simulink model "Controller_HIL"  (R2023b)
settings: Solver=FixedStepDiscrete  StartTime=0.0  StopTime=inf  FixedStep=ts_controller  RelTol=1e-3
InitFcn:
  | mbd_s32k_consistency_checks(bdroot(gcs));
undefined symbols (not defined in the file): Battery, BMS_Controller_State, Charging_State, currentFactor, CV_Gain, DiscIntNeverNeededParam, I_cc, LQFP, MaxCellVoltThrsld, noCurrent, Ns_Module, NumModules, OverCellVoltageLimit, SOCInit, SRE, ts_controller, ts_system, UnderCellVoltageLimit, voltThreshold
libraries: mbd_s32k1xx_ec_toolbox x20, mbd_bcc_ec_toolbox x16, etargetslib x11, simulink x5, sharedTrackingLibrary x2, hdlsllib x1
(part 2 of 2)

== system Controller_HIL/Controller/Controller/SOC Calculation/Measurement Function ==
  Current : Inport
  Temperature (K) : Inport  Port=2
  batteryMeasurementFcn : TriggerPort  TriggerType=function-call  IsSimulinkFunction=on  FunctionName=batteryMeasurementFcn  VariantControl=Variant
  Add1 : Sum  Inputs=+--
  Em Table : Lookup_n-D  BreakpointsForDimension1=Battery.SOC_LUT  BreakpointsForDimension2=Battery.Temperature_LUT  BeginIndexSearchUsingPreviousIndexResult=on  Table=Battery.Em_LUT  ExtrapMethod=Clip  InternalRulePriority=Speed  RndMeth=Simplest
      settings: InputPortMap=u0,u1
  Get SOC : Selector  InputPortWidth=2  IndexOptions=Index vector (dialog)  Indices=[1]  OutputSizes=1
  Get U1 : Selector  InputPortWidth=2  IndexOptions=Index vector (dialog)  Indices=2  OutputSizes=1
  Product : Product
  R0 Table : Lookup_n-D  BreakpointsForDimension1=Battery.SOC_LUT  BreakpointsForDimension2=Battery.Temperature_LUT  BeginIndexSearchUsingPreviousIndexResult=on  Table=Battery.R0_LUT  ExtrapMethod=Clip  InternalRulePriority=Speed  RndMeth=Simplest
      settings: InputPortMap=u0,u1
  x : ArgIn  DisableCoverage=on  OutDataTypeStr=single  PortDimensions=2  ArgumentName=x
  y : ArgOut  DisableCoverage=on  OutDataTypeStr=single  ArgumentName=y
  wires:
  Get U1/1 -> Add1/3  "U1"
  Product/1 -> Add1/2
  Current/1 -> Product/2
  R0 Table/1 -> Product/1
  Temperature (K)/1 -> Em Table/2, R0 Table/2
  Add1/1 -> y/1
  Em Table/1 -> Add1/1
  Get SOC/1 -> Em Table/1, R0 Table/1  "SOC"
  x/1 -> Get SOC/1, Get U1/1

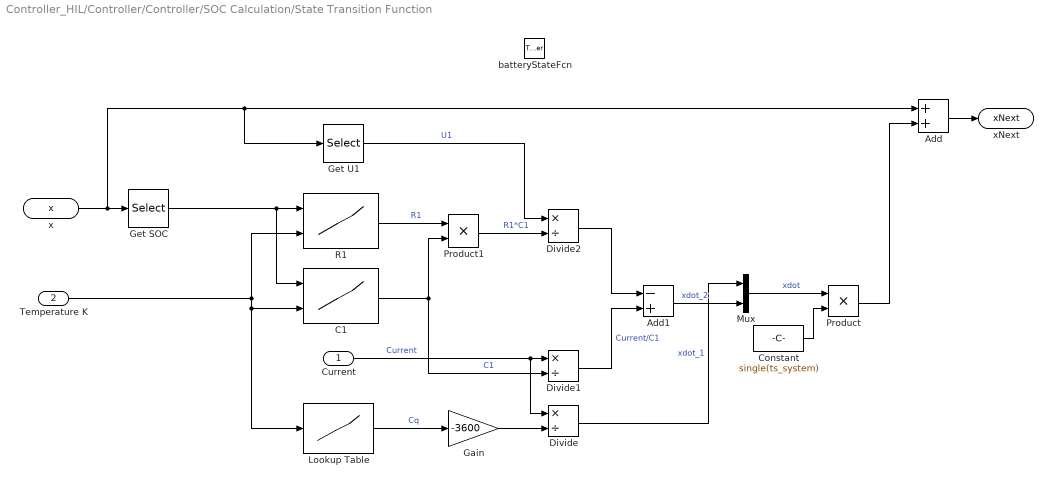
== system Controller_HIL/Controller/Controller/SOC Calculation/State Transition Function ==
  Current : Inport
  Temperature K : Inport  Port=2
  batteryStateFcn : TriggerPort  TriggerType=function-call  IsSimulinkFunction=on  FunctionName=batteryStateFcn  VariantControl=Variant
  Add : Sum
  Add1 : Sum  Inputs=-+
  C1 : Lookup_n-D  BreakpointsForDimension1=Battery.SOC_LUT  BreakpointsForDimension2=Battery.Temperature_LUT  BeginIndexSearchUsingPreviousIndexResult=on  Table=Battery.C1_LUT  ExtrapMethod=Clip  InternalRulePriority=Speed  RndMeth=Simplest
      settings: InputPortMap=u0,u1
  Constant : Constant  Value=single(ts_system)  OutDataTypeStr=single
  Divide : Product  Inputs=*/
  Divide1 : Product  Inputs=*/
  Divide2 : Product  Inputs=*/
  Gain : Gain  Gain=-3600
  Get SOC : Selector  InputPortWidth=2  IndexOptions=Index vector (dialog)  Indices=1  OutputSizes=1
  Get U1 : Selector  InputPortWidth=2  IndexOptions=Index vector (dialog)  Indices=2  OutputSizes=1
  Lookup Table : Lookup_n-D  NumberOfTableDimensions=1  BreakpointsForDimension1=Battery.Temperature_LUT  BeginIndexSearchUsingPreviousIndexResult=on  Table=Battery.Capacity_LUT  InternalRulePriority=Speed  RndMeth=Simplest
  Mux : Mux  Inputs=2
  Product : Product  OutDataTypeStr=single
  Product1 : Product
  R1 : Lookup_n-D  BreakpointsForDimension1=Battery.SOC_LUT  BreakpointsForDimension2=Battery.Temperature_LUT  BeginIndexSearchUsingPreviousIndexResult=on  Table=Battery.R1_LUT  ExtrapMethod=Clip  InternalRulePriority=Speed  RndMeth=Simplest
      settings: InputPortMap=u0,u1
  x : ArgIn  DisableCoverage=on  OutDataTypeStr=single  PortDimensions=2  ArgumentName=x
  xNext : ArgOut  DisableCoverage=on  OutDataTypeStr=single  PortDimensions=2  ArgumentName=xNext
  wires:
  Lookup Table/1 -> Gain/1  "Cq"
  Product/1 -> Add/2
  Constant/1 -> Product/2
  Current/1 -> Divide1/1, Divide/1  "Current"
  Get SOC/1 -> C1/1, R1/1
  Temperature K/1 -> Lookup Table/1, C1/2, R1/2
  Add/1 -> xNext/1
  x/1 -> Add/1, Get U1/1, Get SOC/1
  Gain/1 -> Divide/2
  Divide/1 -> Mux/1  "xdot_1"
  Get U1/1 -> Divide2/1  "U1"
  Product1/1 -> Divide2/2  "R1*C1"
  R1/1 -> Product1/1  "R1"
  C1/1 -> Product1/2, Divide1/2  "C1"
  Divide1/1 -> Add1/2  "Current/C1"
  Divide2/1 -> Add1/1
  Add1/1 -> Mux/2  "xdot_2"
  Mux/1 -> Product/1  "xdot"

== system Controller_HIL/Controller/Controller/SOC Calculation/UKF_EKF_1TC ==
  Cell_Voltage : Inport
  Enable : EnablePort
  EKF : sharedTrackingLibrary/Extended Kalman Filter  StateTransitionFcn=batteryStateFcn  HasStateTransitionJacobianFcn=off  HasAdditiveProcessNoise=Additive  ProcessNoise=1e-10*eye(2)  HasTimeVaryingProcessNoise=off  HasStateTransitionFcnExtraArgument=0  InitialState=[single(SOCInit+0.05); 0;]  InitialStateCovariance=[1e-5 1]  MeasurementFcn1=batteryMeasurementFcn  HasMeasurementJacobianFcn1=off  HasMeasurementEnablePort1=off  HasAdditiveMeasurementNoise1=Additive  MeasurementNoise1=1e-1  HasTimeVaryingMeasurementNoise1=off  HasMeasurementFcnExtraArgument1=0  HasMeasurementWrapping1=off  MeasurementFcn2=myMeasurementFcn  HasMeasurementJacobianFcn2=off  HasMeasurementEnablePort2=off  HasAdditiveMeasurementNoise2=Additive  MeasurementNoise2=1  HasTimeVaryingMeasurementNoise2=off  HasMeasurementFcnExtraArgument2=0  HasMeasurementWrapping2=off  MeasurementFcn3=myMeasurementFcn  HasMeasurementJacobianFcn3=off  HasMeasurementEnablePort3=off  HasAdditiveMeasurementNoise3=Additive  MeasurementNoise3=1  HasTimeVaryingMeasurementNoise3=off  HasMeasurementFcnExtraArgument3=0  HasMeasurementWrapping3=off  MeasurementFcn4=myMeasurementFcn  HasMeasurementJacobianFcn4=off  HasMeasurementEnablePort4=off  HasAdditiveMeasurementNoise4=Additive  MeasurementNoise4=1  HasTimeVaryingMeasurementNoise4=off  HasMeasurementFcnExtraArgument4=0  HasMeasurementWrapping4=off  MeasurementFcn5=myMeasurementFcn  HasMeasurementJacobianFcn5=off  HasMeasurementEnablePort5=off  HasAdditiveMeasurementNoise5=Additive  MeasurementNoise5=1  HasTimeVaryingMeasurementNoise5=off  HasMeasurementFcnExtraArgument5=0  HasMeasurementWrapping5=off  EnableMultirate=off  StateTransitionFcnSampleTime=1  MeasurementFcn1SampleTime=1  MeasurementFcn2SampleTime=1  MeasurementFcn3SampleTime=1  MeasurementFcn4SampleTime=1  MeasurementFcn5SampleTime=1  UseCurrentEstimator=on  OutputStateCovariance=off  DataType=single  SampleTime=ts_controller  NumberOfMeasurements=1
  SOC : Selector  InputPortWidth=2  IndexOptions=Index vector (dialog)  Indices=1  OutputSizes=1
  SOC1 : Selector  InputPortWidth=2  IndexOptions=Index vector (dialog)  Indices=1  OutputSizes=1
  UKF : sharedTrackingLibrary/Unscented Kalman Filter  StateTransitionFcn=batteryStateFcn  HasAdditiveProcessNoise=Additive  ProcessNoise=1e-10*eye(2)  HasTimeVaryingProcessNoise=off  HasStateTransitionFcnExtraArgument=0  InitialState=[single(SOCInit+0.05); 0;]  InitialStateCovariance=[1e-5 1]  Alpha=1  Beta=2  Kappa=1  MeasurementFcn1=batteryMeasurementFcn  HasMeasurementEnablePort1=off  HasAdditiveMeasurementNoise1=Additive  MeasurementNoise1=0.1  HasTimeVaryingMeasurementNoise1=off  HasMeasurementFcnExtraArgument1=0  HasMeasurementWrapping1=off  MeasurementFcn2=myMeasurementFcn  HasMeasurementEnablePort2=off  HasAdditiveMeasurementNoise2=Additive  MeasurementNoise2=1  HasTimeVaryingMeasurementNoise2=off  HasMeasurementFcnExtraArgument2=0  HasMeasurementWrapping2=off  MeasurementFcn3=myMeasurementFcn  HasMeasurementEnablePort3=off  HasAdditiveMeasurementNoise3=Additive  MeasurementNoise3=1  HasTimeVaryingMeasurementNoise3=off  HasMeasurementFcnExtraArgument3=0  HasMeasurementWrapping3=off  MeasurementFcn4=myMeasurementFcn  HasMeasurementEnablePort4=off  HasAdditiveMeasurementNoise4=Additive  MeasurementNoise4=1  HasTimeVaryingMeasurementNoise4=off  HasMeasurementFcnExtraArgument4=0  HasMeasurementWrapping4=off  MeasurementFcn5=myMeasurementFcn  HasMeasurementEnablePort5=off  HasAdditiveMeasurementNoise5=Additive  MeasurementNoise5=1  HasTimeVaryingMeasurementNoise5=off  HasMeasurementFcnExtraArgument5=0  HasMeasurementWrapping5=off  EnableMultirate=off  StateTransitionFcnSampleTime=-1  MeasurementFcn1SampleTime=-1  MeasurementFcn2SampleTime=-1  MeasurementFcn3SampleTime=-1  MeasurementFcn4SampleTime=-1  MeasurementFcn5SampleTime=-1  UseCurrentEstimator=on  OutputStateCovariance=off  DataType=single  SampleTime=ts_controller  NumberOfMeasurements=1
  SOC_UKF : Outport  VectorParamsAs1DForOutWhenUnconnected=off
  SOC_EKF : Outport  Port=2  VectorParamsAs1DForOutWhenUnconnected=off
  wires:
  UKF/1 -> SOC1/1
  Cell_Voltage/1 -> UKF/1, EKF/1
  SOC1/1 -> SOC_UKF/1  "SOC_UKF"
  EKF/1 -> SOC/1
  SOC/1 -> SOC_EKF/1  "SOC_EKF"

== stateflow chart Controller_HIL/Controller/Controller/Balancing Logic/Balancing ==
  settings: updateMethod=DISCRETE
  state BalancingOFF
    en:
    Bal_Cmd(:,:) = false;
    en,du:
    MaxCellVolt = max(CellVoltages);
    MinCellVolt = min(CellVoltages);
    DeltaCellVolt = MaxCellVolt - MinCellVolt;
  state BalancingON
    en, du:
    MaxCellVolt = max(CellVoltages);
    MinCellVolt = min(CellVoltages);
    DeltaCellVolt = MaxCellVolt - MinCellVolt;
    state BalActive
      en, du:
      Bal_Cmd = ((CellVoltages - MinCellVolt) > TargetDeltaV)';
      flgBalCompl = all(~Bal_Cmd);
    state BalNotActive
    (default) -> BalActive
    BalNotActive -> BalActive [order 1] : [after(BalNotActWait,sec) && ...
        | DeltaCellVolt > TargetDeltaV]
    BalActive -> BalNotActive : [flgBalCompl]
  note: "Copyright 2018 - 2019 The MathWorks, Inc."
  (default) -> BalancingOFF : {flgBalCompl = true;}
  BalancingOFF -> BalancingON : [flgEnBalancing && ...
      | BMS_State ~= BMS_Controller_State.BMS_Driving && ...
      | BMS_State ~= BMS_Controller_State.BMS_Fault && ...
      | after(BalOffWait,sec) && ...
      | DeltaCellVolt > TargetDeltaV]
  BalancingON -> BalancingOFF : [BMS_State == BMS_Controller_State.BMS_Driving]
  BalNotActive -> BalancingOFF [order 2] : [after(BalOnWait,sec)]
  data: BMS_State input Enum: BMS_Controller_State; CellVoltages input single; Bal_Cmd output boolean size=[1,Ns_Module*NumModules] =boolean(zeros(1,Ns_Module*NumModules)); flgBalCompl local; BalNotActWait local =int16(10); BalOffWait local =int16(5); BalOnWait local =int16(20); flgEnBalancing local =boolean(1); DeltaCellVolt local single =single(0); MaxCellVolt local =single(4); MinCellVolt local =single(3); TargetDeltaV local =single(0.1)

== matlab function Controller_HIL/Controller/Controller/SOC Calculation/MATLAB Function ==
  data: meas input double; xhatOut output double
function xhatOut  = EXTKALMAN(meas)
%EXTKALMAN Radar Data Processing Tracker Using an Extended Kalman Filter
%
%  This program is executed as a MATLAB function block in the 
%  sldemo_radar Simulink model.  The estimated and actual positions are 
%  saved to the workspace and are plotted at the end of the simulation by 
%  the program aero_radplot (called from the simulation automatically).
%
%

%  Copyright 1990-2013 The MathWorks, Inc.
deltat = 0.1;
% Initialization
persistent P;
persistent xhat
if isempty(P)
    xhat = [0.75; 0];
    P = 1e-10*eye(2);
end
    
%  Radar update time deltat is inherited from model workspace

% 1. Compute Phi, Q, and R 
Phi = [1 deltat; 0 1];
%Phi = deltat;
Q =  1e-10*eye(2);
R =  1e-1;

% 2. Propagate the covariance matrix:
P = Phi*P*Phi' + Q;

% 3. Propagate the track estimate::
xhat = Phi*xhat;

% 4 a). Compute observation estimates:
xNext = batteryStateFnc(xhat);

% 4 b). Compute observation vector y and linearized measurement matrix M 
yhat = batteryMeasurementFcn(xhat);
M = [ cos(xNext(1))          0 sin(xNext(1))          0
   -sin(xNext(1))/xNext(2) 0 cos(xNext(1))/xNext(2) 0 ];
% 4 c).  Compute residual (Estimation Error)
residual = meas - yhat;

% 5. Compute Kalman Gain:
W = P*M'*inv(M*P*M'+ R);

% 6. Update estimate
xhat = xhat + W*residual;

% 7. Update Covariance Matrix
P = (eye(4)-W*M)*P*(eye(4)-W*M)' + W*R*W';

xhatOut = xhat;

== stateflow chart Controller_HIL/Controller/Controller/BMS State Machine/State_Machine ==
  settings: updateMethod=DISCRETE  sampleTime=ts_controller
  state MainStateMachine [parallel]
    settings: executionOrder=1
    state Standby
      en:
      BMS_State = ...
      BMS_Controller_State.BMS_Idle;
    state Charging
      en:
      BMS_State = BMS_Controller_State.BMS_Charging;
      state Init_Mode
        en:
        ChargeModeReq = Charging_State.Init;
        ChargeCurrentReq = noCurrent;
      state CC_Mode
        en:
        ChargeModeReq = Charging_State.CC;
        du:
        ChargeCurrentReq = min(I_cc,ChargeCurrentLimit);
      state CV_Mode
        en:
        ChargeModeReq = Charging_State.CV;
        du:
        ChargeCurrentReq = ChargeCurrentReq - CV_Gain*(MaxCellVolt - MaxCellVoltThrsld);
        ChargeCurrentReq = min(ChargeCurrentReq, ChargeCurrentLimit);
      (default) -> Init_Mode
      CV_Mode -> Init_Mode : [State_Request ~= SRE.Charging || ...
          | ChargeCurrentReq <= (I_cc/currentFactor)]
      CC_Mode -> Init_Mode [order 1] : [State_Request ~= ...
          | SRE.Charging]
      Init_Mode -> CC_Mode : [State_Request == SRE.Charging && ...
          | MaxCellVolt < voltThreshold]
      CC_Mode -> CV_Mode [order 2] : [MaxCellVolt>=...
          | MaxCellVoltThrsld]
    state Driving
      en:
      BMS_State = ...
      BMS_Controller_State.BMS_Driving;
    state Fault
      en,du:
      BMS_State = ...
      BMS_Controller_State.BMS_Fault;
    (default) -> Standby
    Standby -> Fault [order 1] : [FaultPresent == true]
    Standby -> Charging [order 2] : [State_Request == SRE.Charging]
    (junction 699) -> Standby : [after(3,sec)]
    Charging -> Standby [order 3] : [State_Request ~= SRE.Charging]
    Standby -> Driving [order 3] : [State_Request == SRE.Driving]
    Driving -> Standby [order 3] : [State_Request ~= SRE.Driving]
    Driving -> Charging [order 2] : [State_Request == SRE.Charging]
    Charging -> Driving [order 2] : [State_Request == SRE.Driving]
    Fault -> (junction 699) : [[FaultPresent == false && Fault_Reset_Enable]]
    Driving -> Fault [order 1] : [FaultPresent]
    Charging -> Fault [order 1] : [FaultPresent]{ChargeCurrentReq = single(0);}
  state FaultMonitoring [parallel]
    settings: executionOrder=2
    state MonitorCellVoltage [parallel]
      settings: executionOrder=1
      state OverVoltageFault
        en:
        FaultPresent = true;
        Fault_out.OverVolt = true;
        du:
        MaxCellVolt = max(Cell_Voltages);
      state NoCellVoltFault
        en,du:
        MaxCellVolt = max(Cell_Voltages);
        MinCellVolt = min(Cell_Voltages);
      state UnderVoltageFault
        en:
        FaultPresent = true;
        Fault_out.UnderVolt = true;
        du:
        MinCellVolt = min(Cell_Voltages);
      OverVoltageFault -> (junction 687) : [MaxCellVolt < OverCellVoltageLimit && ...
          | Fault_Reset_Enable ...
          | ]{Fault_out.OverVolt=false; ...
          | FaultPresent = false;}
      (junction 695) -> OverVoltageFault : [after(100,msec)]
      NoCellVoltFault -> (junction 695) [order 1] : [MaxCellVolt >= ...
          | OverCellVoltageLimit]
      (junction 687) -> NoCellVoltFault : [after(3,sec)]
      (default) -> NoCellVoltFault : {FaultPresent = false;
          | Fault_out.OverVolt = false;
          | Fault_out.UnderVolt = false;}
      NoCellVoltFault -> (junction 697) [order 2] : [MinCellVolt <=...
          |  UnderCellVoltageLimit]
      (junction 685) -> NoCellVoltFault : [after(3,sec)]
      (junction 697) -> UnderVoltageFault : [after(100,msec)]
      UnderVoltageFault -> (junction 685) : [MinCellVolt > UnderCellVoltageLimit && ...
          | Fault_Reset_Enable] ...
          | {Fault_out.UnderVolt=false; ...
          | FaultPresent = false;}
    state MonitorCurrLim [parallel]
      settings: executionOrder=3
      state NoCurrLimFault
        en:
        FaultPresent = false;
        Fault_out.OverCurrent = false;
      state OverCurrentFault
        en:
        FaultPresent = true;
        Fault_out.OverCurrent=true;
      (default) -> NoCurrLimFault : {FaultPresent = false;
          | Fault_out.OverCurrent=false;}
      (junction 678) -> NoCurrLimFault : [after(3,sec)]
      NoCurrLimFault -> (junction 675) : [((DischargeCurrentLimit - Pack_Current) > single(0.2) && ...
          | BMS_State == BMS_Controller_State.BMS_Driving) || ...
          | ((Pack_Current - ChargeCurrentLimit) > single(0.2) && ...
          | BMS_State == BMS_Controller_State.BMS_Charging)]
      OverCurrentFault -> (junction 678) : [(Pack_Current >= DischargeCurrentLimit || ...
          |  Pack_Current <= ChargeCurrentLimit) && ...
          | Fault_Reset_Enable]
      (junction 675) -> OverCurrentFault : [after(100,msec)]
    state MonitorCellTemp [parallel]
      settings: executionOrder=2
      state HighTemperatureFault
        en:
        FaultPresent = true;
        Fault_out.HighTemp = true;
        du:
        MaxCellTemp = max(Cell_Temperatures);
      state NoCellTempFault
        en,du:
        MaxCellTemp = max(Cell_Temperatures);
        MinCellTemp = min(Cell_Temperatures);
      state LowTemperatureFault
        en:
        FaultPresent = true;
        Fault_out.LowTemp = true;
        du:
        MinCellTemp = min(Cell_Temperatures);
      HighTemperatureFault -> (junction 680) : [MaxCellTemp < HighTempLimit && ...
          | Fault_Reset_Enable] ...
          | {Fault_out.HighTemp=false; FaultPresent = false;}
      (junction 689) -> HighTemperatureFault : [after(100,msec)]
      (junction 680) -> NoCellTempFault : [after(3,sec)]
      NoCellTempFault -> (junction 689) [order 1] : [MaxCellTemp >= HighTempLimit]
      (default) -> NoCellTempFault : {FaultPresent = false;
          | Fault_out.HighTemp = false;
          | Fault_out.LowTemp = false;}
      (junction 682) -> NoCellTempFault : [after(3,sec)]
      NoCellTempFault -> (junction 691) [order 2] : [MinCellTemp <= LowTempLimit]
      LowTemperatureFault -> (junction 682) : [MinCellTemp > LowTempLimit && ...
          | Fault_Reset_Enable ] ...
          | {Fault_out.LowTemp=false; FaultPresent = false;}
      (junction 691) -> LowTemperatureFault : [after(100,msec)]
  data: DischargeCurrentLimit input single; ChargeCurrentLimit input single; State_Request input; Cell_Voltages input single; Pack_Voltage input single; Cell_Temperatures input single; Pack_Current input single; ChargeCurrentReq output; I_cc parameter; MaxCellVoltThrsld parameter; FaultPresent local; MaxCellTemp local; OverCellVoltageLimit parameter; UnderCellVoltageLimit parameter; MinCellTemp local; CV_Gain parameter; MonitorCurrLimMode local Enum: MonitorCurrLimModeType; MonitorCellVoltageMode local Enum: MonitorCellVoltageModeType; MonitorCellTempMode local Enum: MonitorCellTempModeType; Fault_out output Bus: Faults; voltThreshold parameter single; currentFactor parameter single; noCurrent parameter single; Fault_Reset_Enable input boolean; ChargeModeReq output Enum: Charging_State =Charging_State.Init; BMS_State output Enum: BMS_Controller_State =BMS_Controller_State.BMS_Idle; MaxCellVolt local; MinCellVolt local; HighTempLimit local =single(323.15); LowTempLimit local =single(278.15)
